simulink model "VCU_Software_Harness2"  (R2024a)
settings: Solver=FixedStepDiscrete  StartTime=0  StopTime=150  FixedStep=0.01  RelTol=2e-1  AbsTol=1e-1
undefined symbols (not defined in the file): Drv_Mode
libraries: SignalEditorBlockLib x1
settings Model: DataDictionary=VirtualVehicleTemplate.sldd  Creator=smuckati  LastModifiedBy=smuckati
settings SolverCC: AutoScaleAbsTol=off  SolverJacobianMethodControl=FullPerturbation  ZeroCrossAlgorithm=Adaptive  AlgebraicLoopSolver=TrustRegion  AutoInsertRateTranBlk=on  InsertRTBMode=Never (minimum delay)  DecoupledContinuousIntegration=on  MinimalZcImpactIntegration=on  MaxZcPerStep=1
settings OptimizationCC: DefaultParameterBehavior=Inlined  UseDivisionForNetSlopeComputation=on  GainParamInheritBuiltInType=on  UseFloatMulNetSlope=on  UseSpecifiedMinMax=on  InlineInvariantSignals=on  BitwiseOrLogicalOp=Bitwise operator  PassReuseOutputArgsAs=Individual arguments  ZeroExternalMemoryAtStartup=off  ZeroInternalMemoryAtStartup=off  NoFixptDivByZeroProtection=on  EfficientFloat2IntCast=on  LifeSpan=1  OptimizeBlockOrder=speed  DifferentSizesBufferReuse=on  EfficientTunableParamExpr=on
settings DebuggingCC: SignalInfNanChecking=error  ArtificialAlgebraicLoopMsg=none  MaskedZcDiagnostic=none  IgnoredZcDiagnostic=none  ParameterTunabilityLossMsg=error  UnconnectedInputMsg=warning  UnconnectedOutputMsg=warning  UnconnectedLineMsg=warning  PregeneratedLibrarySubsystemCodeDiagnostic=none  SubsystemReferenceDiagnosticForUnitTest=warning  ArithmeticOperatorsInVariantConditions=warning
settings HardwareCC: ProdBitPerPointer=32  ProdBitPerSizeT=32  ProdBitPerPtrDiffT=32  ProdLargestAtomicFloat=None  ProdWordSize=32  ProdHWDeviceType=Custom Processor->Custom Processor
settings ModelReferenceCC: UpdateModelReferenceTargets=IfOutOfDate  EnableRefExpFcnMdlSchedulingChecks=on  ModelReferenceMinAlgLoopOccurrences=on  PropagateSignalLabelsOutOfModel=off
settings SFSimCC: SimUseLocalCustomCode=off  SimGenImportedTypeDefs=on  MATLABDynamicMemAlloc=off  SimTargetLang=C++
settings RTWCC: Description=AUTOSAR Adaptive  SystemTargetFile=autosar_adaptive.tlc  GenCodeOnly=on  PackageGeneratedCodeAndArtifacts=on  TemplateMakefile=ert_default_tmf  GenerateReport=on  RTWUseLocalCustomCode=off  Toolchain=AUTOSAR Adaptive | CMake  BuildConfiguration=Faster Runs  IncludeHyperlinkInReport=on  DataTypeReplacement=CDataTypesFixedWidth  TargetLang=C++  GenerateTraceInfo=on  GenerateTraceReport=on  GenerateTraceReportSl=on  GenerateTraceReportSf=on  GenerateTraceReportEml=on  GenerateCodeMetricsReport=on  GenerateCodeReplacementReport=on  GPUComputeCapability=3.5  DLArmComputeVersion=19.05
settings CodeAppCC: ForceParamTrailComments=on  IgnoreCustomStorageClasses=off  MaxIdLength=63  OperatorAnnotations=on  SimulinkDataObjDesc=on  SFDataObjDesc=on  CustomSymbolStrGlobalVar=rt$N$M  CustomSymbolStrType=$N$M  CustomSymbolStrFcn=$N$M$F  CustomSymbolStrMacro=$N$M  InsertBlockDesc=on
settings AUTOSARAdaptiveTargetCC: TargetFcnLib=ansi_tfl_table_tmw.mat  GenFloatMathFcnCalls=NOT IN USE  TargetLangStandard=C++11 (ISO)  CodeReplacementLibrary=C++ Standard Library Mutex  UtilityFuncGeneration=Auto  MultiwordTypeDef=System defined  MultiwordLength=2048  DynamicStringBufferSize=256  GenerateFullHeader=on  InferredTypesCompatibility=off  GenerateSampleERTMain=off  GenerateTestInterfaces=off  ModelReferenceCompliant=on  ParMdlRefBuildCompliant=on  CompOptLevelCompliant=on  ConcurrentExecutionCompliant=on  IncludeMdlTerminateFcn=on  CombineOutputUpdateFcns=on  CombineSignalStateStructs=on  GroupInternalDataByFunction=off  SuppressErrorStatus=on  IncludeFileDelimiter=Auto  ERTCustomFileBanners=off  SupportAbsoluteTime=off  LogVarNameModifier=rt_  MatFileLogging=off  CodeInterfacePackaging=C++ class  PurelyIntegerCode=off  SupportNonFinite=off  SupportComplex=off  SupportContinuousTime=off  SupportNonInlinedSFcns=off  RemoveDisableFunc=off  RemoveResetFunc=on  SupportVariableSizeSignals=off  ParenthesesLevel=Nominal  CastingMode=Nominal  MATLABClassNameForMDSCustomization=Simulink.SoftwareTarget.TargetSpecificTriggerConfigurationBase  ModelStepFunctionPrototypeControlCompliant=off  CPPClassGenCompliant=on  AutosarCompliant=on  MDXCompliant=off  GRTInterface=off  GenerateAllocFcn=off  UseToolchainInfoCompliant=on  GenerateSharedConstants=on  CoderGroups=[]  AccessMethods=[]  LookupTableObjectStructAxisOrder=2,1,3,4,...  LUTObjectStructOrderExplicitValues=Size,Breakpoints,Table  LUTObjectStructOrderEvenSpacing=Size,Table,Breakpoints  ArrayLayout=Column-major  UnsupportedSFcnMsg=error  ERTHeaderFileRootName=$R$E  ERTSourceFileRootName=$R$E  ERTDataFileRootName=$R_data  InstructionSetFMA=off  OptimizeReductions=off  LogToMDFFile=off  GenerateASAP2=off  DSAsUniqueAccess=off  ExtMode=off  ExtModeTransport=0  ExtModeStaticAlloc=off  ExtModeAutomaticAllocSize=on  ExtModeMaxTrigDuration=10  ExtModeStaticAllocSize=1000000  ExtModeTesting=off  ExtModeMexFile=ext_comm  ExtModeIntrfLevel=Level1  InlinedParameterPlacement=NonHierarchical  TargetOS=BareBoardExample  MultiInstanceErrorCode=Error  RootIOFormat=Structure reference  RTWCAPISignals=off  RTWCAPIParams=off  RTWCAPIStates=off  RTWCAPIRootIO=off  ERTSrcFileBannerTemplate=ert_code_template.cgt  ERTHdrFileBannerTemplate=ert_code_template.cgt  ERTDataSrcFileTemplate=ert_code_template.cgt  ERTDataHdrFileTemplate=ert_code_template.cgt  ERTCustomFileTemplate=example_file_process.tlc  EnableDataOwnership=off  SignalDisplayLevel=10  ParamTuneLevel=10  GlobalDataDefinition=Auto  DataDefinitionFile=global.c  GlobalDataReference=Auto  ERTFilePackagingFormat=CompactWithDataFile  RateTransitionBlockCode=Inline  DataReferenceFile=global.h  PreserveExpressionOrder=off  PreserveIfCondition=off  ConvertIfToSwitch=on  PreserveExternInFcnDecls=on  PreserveStaticInFcnDecls=on  SuppressUnreachableDefaultCases=on  EnableSignedLeftShifts=on  EnableSignedRightShifts=on  ImplementImageWithCVMat=off  IndentStyle=K&R  IndentSize=2  NewlineStyle=Default  MaxLineWidth=80  EnableUserReplacementTypes=off  MaxIdInt64=INT64_MAX  MinIdInt64=INT64_MIN  MaxIdUint64=UINT64_MAX  MaxIdInt32=INT32_MAX  MinIdInt32=INT32_MIN  MaxIdUint32=UINT32_MAX  MaxIdInt16=INT16_MAX  MinIdInt16=INT16_MIN  MaxIdUint16=UINT16_MAX  MaxIdInt8=INT8_MAX  MinIdInt8=INT8_MIN  MaxIdUint8=UINT8_MAX  BooleanTrueId=true  BooleanFalseId=false  MemSecPackage=--- None ---  MemSecDataConstants=Default  MemSecDataIO=Default  MemSecDataInternal=Default  MemSecDataParameters=Default  MemSecFuncInitTerm=Default  MemSecFuncExecute=Default  MemSecFuncSharedUtil=Default  GroupConstants=Default  GroupRootInputs=Default  GroupRootOutputs=Default  GroupInternal=Default  GroupParameters=Default  GroupDataTransfer=Default  GroupSharedLocalDataStores=Default  GroupInstanceSpecificParameters=Default  GroupModelData=Default  ArrayContainerType=std::array  AutosarSchemaVersion=R20-11  AutosarMaxShortNameLength=128  AdaptiveAutosarXCPServerTransportLayer=None  AdaptiveAutosarXCPServerTCPIPAddress=127.0.0.1  AdaptiveAutosarXCPServerPort=17725  AdaptiveAutosarXCPServerVerbosity=off  AdaptiveAutosarUseCustomXCPServer=off

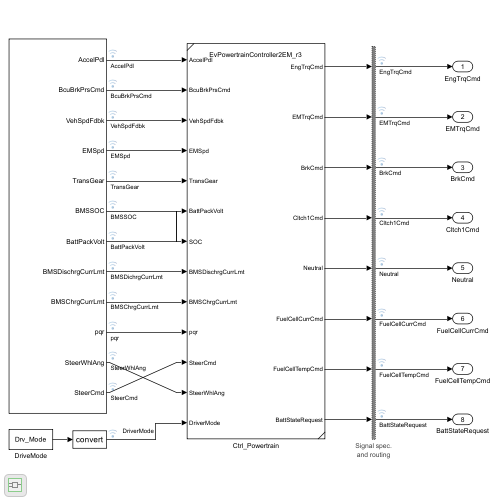
[thumbnail: Simulink's stored preview of the top-level diagram]
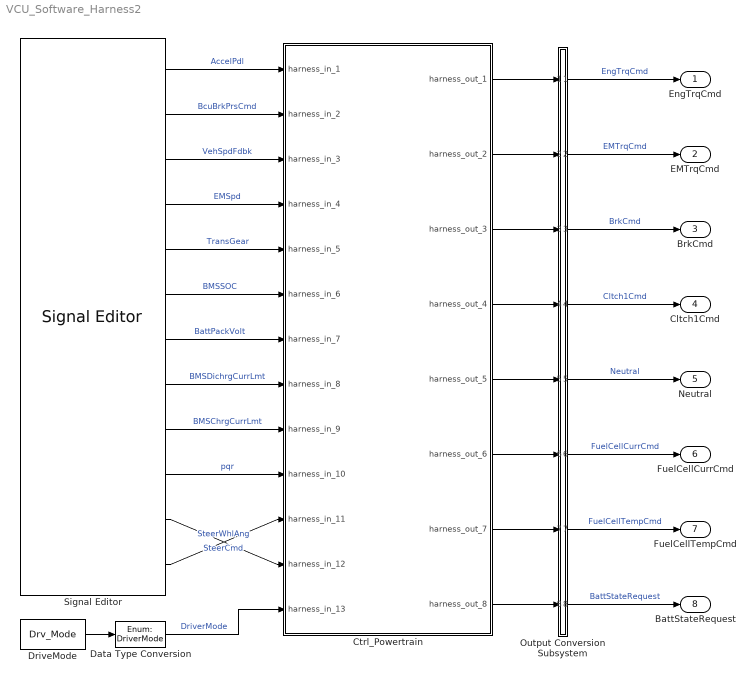
== system VCU_Software_Harness2 ==
  Ctrl_Powertrain : Subsystem  Tag=__SL_testing_harness_stub_
  Data Type Conversion : DataTypeConversion  OutDataTypeStr=Enum: DriverMode  SaturateOnIntegerOverflow=off  RndMeth=Floor
  DriveMode : Constant  Value=Drv_Mode  OutDataTypeStr=int8
  Output Conversion Subsystem : Subsystem  Tag=__SLT_OCS__  Description=|
      | Signal spec.
      | and routing
      settings: AttributesFormatString=%<Description>
  Signal Editor : SignalEditorBlockLib/Signal Editor  FileName=VCU_Inpts.mat  ActiveScenario=Scenario1  ActiveSignal=SteerCmd  IsBus=off  OutputBusObjectStr=Bus: BusObject  SampleTime=0.01  Interpolate=off  ZeroCross=off  OutputAfterFinalValue=Setting to zero  Unit=inherit  PreserveSignalName=on  ApplySigPropsToAllScenarios=on  ApplySigPropsToAllSignals=off
  EngTrqCmd : Outport
  EMTrqCmd : Outport  Port=2
  BrkCmd : Outport  Port=3
  Cltch1Cmd : Outport  Port=4
  Neutral : Outport  Port=5
  FuelCellCurrCmd : Outport  Port=6
  FuelCellTempCmd : Outport  Port=7
  BattStateRequest : Outport  Port=8
  wires:
  Output Conversion Subsystem/1(Outport_1) -> EngTrqCmd/1  "EngTrqCmd"
  Output Conversion Subsystem/2(Outport_2) -> EMTrqCmd/1  "EMTrqCmd"
  Output Conversion Subsystem/3(Outport_3) -> BrkCmd/1  "BrkCmd"
  Output Conversion Subsystem/4(Outport_4) -> Cltch1Cmd/1  "Cltch1Cmd"
  Output Conversion Subsystem/5(Outport_5) -> Neutral/1  "Neutral"
  Output Conversion Subsystem/6(Outport_6) -> FuelCellCurrCmd/1  "FuelCellCurrCmd"
  Output Conversion Subsystem/7(Outport_7) -> FuelCellTempCmd/1  "FuelCellTempCmd"
  Output Conversion Subsystem/8(Outport_8) -> BattStateRequest/1  "BattStateRequest"
  Ctrl_Powertrain/1(harness_out_1) -> Output Conversion Subsystem/1(Inport_1)
  Ctrl_Powertrain/2(harness_out_2) -> Output Conversion Subsystem/2(Inport_2)
  Ctrl_Powertrain/3(harness_out_3) -> Output Conversion Subsystem/3(Inport_3)
  Ctrl_Powertrain/4(harness_out_4) -> Output Conversion Subsystem/4(Inport_4)
  Ctrl_Powertrain/5(harness_out_5) -> Output Conversion Subsystem/5(Inport_5)
  Ctrl_Powertrain/6(harness_out_6) -> Output Conversion Subsystem/6(Inport_6)
  Ctrl_Powertrain/7(harness_out_7) -> Output Conversion Subsystem/7(Inport_7)
  Ctrl_Powertrain/8(harness_out_8) -> Output Conversion Subsystem/8(Inport_8)
  DriveMode/1 -> Data Type Conversion/1
  Signal Editor/5 -> Ctrl_Powertrain/5(harness_in_5)  "TransGear"
  Data Type Conversion/1 -> Ctrl_Powertrain/13(harness_in_13)  "DriverMode"
  Signal Editor/3 -> Ctrl_Powertrain/3(harness_in_3)  "VehSpdFdbk"
  Signal Editor/7 -> Ctrl_Powertrain/7(harness_in_7)  "BattPackVolt"
  Signal Editor/8 -> Ctrl_Powertrain/8(harness_in_8)  "BMSDichrgCurrLmt"
  Signal Editor/6 -> Ctrl_Powertrain/6(harness_in_6)  "BMSSOC"
  Signal Editor/10 -> Ctrl_Powertrain/10(harness_in_10)  "pqr"
  Signal Editor/1 -> Ctrl_Powertrain/1(harness_in_1)  "AccelPdl"
  Signal Editor/2 -> Ctrl_Powertrain/2(harness_in_2)  "BcuBrkPrsCmd"
  Signal Editor/9 -> Ctrl_Powertrain/9(harness_in_9)  "BMSChrgCurrLmt"
  Signal Editor/4 -> Ctrl_Powertrain/4(harness_in_4)  "EMSpd"
  Signal Editor/11 -> Ctrl_Powertrain/12(harness_in_12)  "SteerWhlAng"
  Signal Editor/12 -> Ctrl_Powertrain/11(harness_in_11)  "SteerCmd"

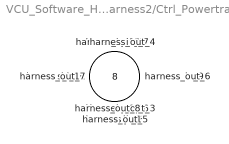
== system VCU_Software_Harness2/Ctrl_Powertrain ==
  harness_in_1 : Inport
  harness_in_2 : Inport  Port=2
  harness_in_3 : Inport  Port=3
  harness_in_4 : Inport  Port=4
  harness_in_5 : Inport  Port=5
  harness_in_6 : Inport  Port=6
  harness_in_7 : Inport  Port=7
  harness_in_8 : Inport  Port=8
  harness_in_9 : Inport  Port=9
  harness_in_10 : Inport  Port=10
  harness_in_11 : Inport  Port=11
  harness_in_12 : Inport  Port=12
  harness_in_13 : Inport  Port=13
  harness_out_1 : Outport
  harness_out_2 : Outport  Port=2
  harness_out_3 : Outport  Port=3
  harness_out_4 : Outport  Port=4
  harness_out_5 : Outport  Port=5
  harness_out_6 : Outport  Port=6
  harness_out_7 : Outport  Port=7
  harness_out_8 : Outport  Port=8

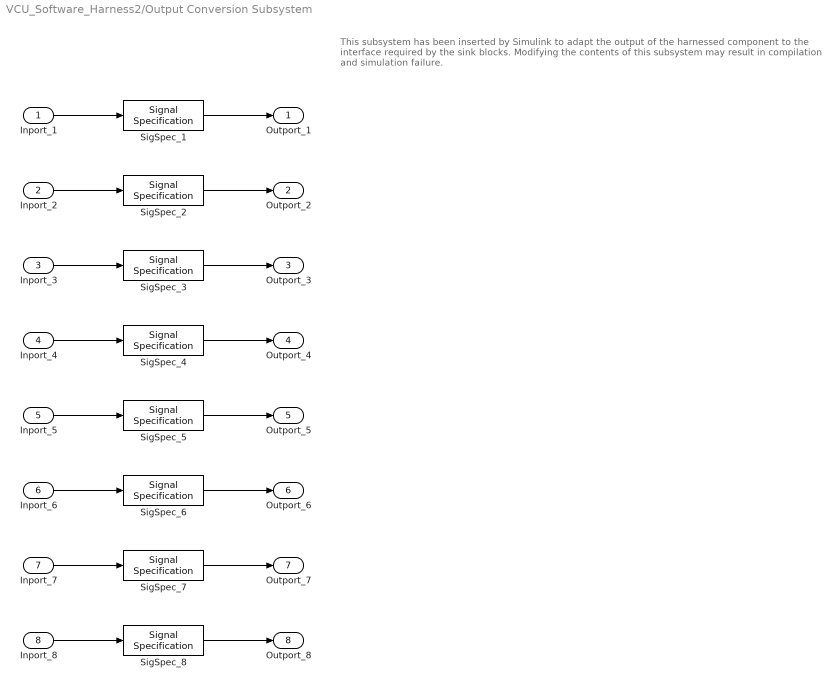
== system VCU_Software_Harness2/Output Conversion Subsystem ==
  note: This subsystem has been inserted by Simulink to adapt the output of the harnessed component to the interface required by the sink blocks.
      |  Modifying the contents of this subsystem may result in compilation and simulation failure.
  Inport_1 : Inport
  Inport_2 : Inport  Port=2
  Inport_3 : Inport  Port=3
  Inport_4 : Inport  Port=4
  Inport_5 : Inport  Port=5
  Inport_6 : Inport  Port=6
  Inport_7 : Inport  Port=7
  Inport_8 : Inport  Port=8
  SigSpec_{1,4..7} (5 alike) : SignalSpecification  OutDataTypeStr=double  Dimensions=[1]  SampleTime=0.01
  SigSpec_2 : SignalSpecification  OutDataTypeStr=double  Dimensions=[2]  SampleTime=0.01
  SigSpec_3 : SignalSpecification  OutDataTypeStr=double  Dimensions=[4]  SampleTime=0.01
  SigSpec_8 : SignalSpecification  OutDataTypeStr=Enum: SRE  Dimensions=[1]  SampleTime=0.01
  Outport_1 : Outport
  Outport_2 : Outport  Port=2
  Outport_3 : Outport  Port=3
  Outport_4 : Outport  Port=4
  Outport_5 : Outport  Port=5
  Outport_6 : Outport  Port=6
  Outport_7 : Outport  Port=7
  Outport_8 : Outport  Port=8
  wires:
  Inport_1/1 -> SigSpec_1/1
  SigSpec_1/1 -> Outport_1/1
  Inport_2/1 -> SigSpec_2/1
  SigSpec_2/1 -> Outport_2/1
  Inport_3/1 -> SigSpec_3/1
  SigSpec_3/1 -> Outport_3/1
  Inport_4/1 -> SigSpec_4/1
  SigSpec_4/1 -> Outport_4/1
  Inport_5/1 -> SigSpec_5/1
  SigSpec_5/1 -> Outport_5/1
  Inport_6/1 -> SigSpec_6/1
  SigSpec_6/1 -> Outport_6/1
  Inport_7/1 -> SigSpec_7/1
  SigSpec_7/1 -> Outport_7/1
  Inport_8/1 -> SigSpec_8/1
  SigSpec_8/1 -> Outport_8/1
